simulink model "psbcontrolvolt"  (Simulink 6.0)
settings: Solver=ode23tb  SolverMode=SingleTasking  StartTime=0.0  StopTime=0.1  MaxStep=1e-04  RelTol=1e-3  AbsTol=1e-6
InitFcn:
  | powericon('psbinitsys',bdroot);
libraries: powerlib2 x12
settings Model: Creator=patrice  LastModifiedBy=batserve  ExtModeTrigMode=oneshot  ExtModeArmWhenConnect=off  ExtModeAutoUpdateStatusClock=off
settings DataIOCC: LimitDataPoints=off  SignalLoggingName=sigsOut
settings OptimizationCC: BlockReduction=off  BooleanDataType=off
settings DebuggingCC: SolverPrmCheckMsg=none
settings HardwareCC: TargetUnknown=on
settings RTWCC: TemplateMakefile=grt_unix.tmf

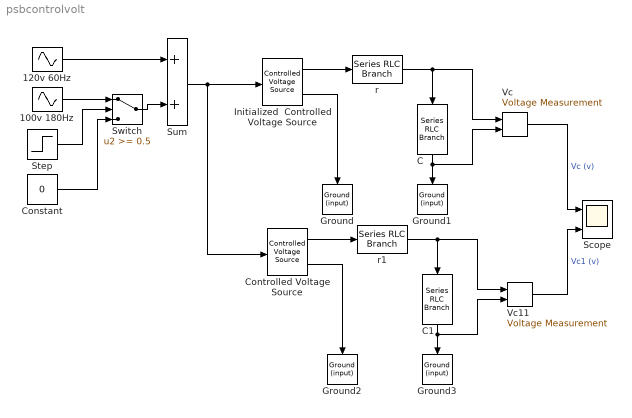
== system psbcontrolvolt ==
  100v 180Hz : Sin  Amplitude=100  Frequency=2*pi*180  SampleTime=0
  120v 60Hz : Sin  Amplitude=120  Frequency=2*pi*60  SampleTime=0
  C : powerlib2/Elements/Series RLC Branch  Tag=PoWeRsYsTeMbLoCk  Orientation=down  a=0  b=0  c=500e-6  mesure=None  PSBOutputType=1
  C1 : powerlib2/Elements/Series RLC Branch  Tag=PoWeRsYsTeMbLoCk  Orientation=down  a=0  b=0  c=500e-6  mesure=None  PSBOutputType=1
  Constant : Constant  Value=0
  Controlled Voltage Source : powerlib2/Electrical Sources/Controlled Voltage Source  Tag=PoWeRsYsTeMbLoCk  initsrc=off  srctyp=AC  iv=120  iph=0  ifreq=60  mesure=None  PSBOutputType=11
  Ground{,1..3} (4 alike) : powerlib2/Connectors/Ground (input)  Tag=PoWeRsYsTeMbLoCk  Orientation=down
  Initialized  Controlled Voltage Source : powerlib2/Electrical Sources/Controlled Voltage Source  Tag=PoWeRsYsTeMbLoCk  initsrc=on  srctyp=AC  iv=120  iph=0  ifreq=60  mesure=None  PSBOutputType=11
  Scope : Scope  NumInputPorts=2
      settings: TickLabels=on  TimeRange=0.1  YMin=-100~-100  YMax=100~100  DataFormat=Array
  Step : Step  Time=2/60  SampleTime=0
  Sum : Sum  SaturateOnIntegerOverflow=on  InputSameDT=on
  Switch : Switch  Threshold=0.5  SaturateOnIntegerOverflow=on  InputSameDT=on
  Vc : powerlib2/Measurements/Voltage Measurement  Tag=PoWeRsYsTeMmEaSuReMeNt  PhasorSimulation=off  OutputType=Magnitude  PSBOutputType=0  PSBequivalent=0
  Vc11 : powerlib2/Measurements/Voltage Measurement  Tag=PoWeRsYsTeMmEaSuReMeNt  PhasorSimulation=off  OutputType=Magnitude  PSBOutputType=0  PSBequivalent=0
  r : powerlib2/Elements/Series RLC Branch  Tag=PoWeRsYsTeMbLoCk  a=10  b=0  c=inf  mesure=None  PSBOutputType=1
  r1 : powerlib2/Elements/Series RLC Branch  Tag=PoWeRsYsTeMbLoCk  a=10  b=0  c=inf  mesure=None  PSBOutputType=1
  wires:
  Initialized  Controlled Voltage Source/2 -> Ground/1
  Vc/1 -> Scope/1  "Vc (v)"
  120v 60Hz/1 -> Sum/1
  Switch/1 -> Sum/2
  Step/1 -> Switch/2
  100v 180Hz/1 -> Switch/1
  Constant/1 -> Switch/3
  Initialized  Controlled Voltage Source/1 -> r/1
  r/1 -> C/1, Vc/1
  C/1 -> Ground1/1, Vc/2
  Vc11/1 -> Scope/2  "Vc1 (v)"
  Sum/1 -> Initialized  Controlled Voltage Source/1, Controlled Voltage Source/1
  Controlled Voltage Source/2 -> Ground2/1
  Controlled Voltage Source/1 -> r1/1
  r1/1 -> Vc11/1, C1/1
  C1/1 -> Vc11/2, Ground3/1
